simulink model "XMC_DSPLib_Solution_Stage1"  (R2020a)
settings: Solver=VariableStepAuto  StartTime=0.0  StopTime=5000  RelTol=1e-3
PreLoadFcn:
  | CreateFilter;
InitFcn:
  | CreateFilter;
undefined symbols (not defined in the file): cfi, hb1, hb2, hb3, Shift1, Shift2, Shift3, ShiftCF
libraries: ModelComposer x5, dspmlti4 x3, dspsrcs4 x1
settings Model: Creator=oliviert  LastModifiedBy=oliviert

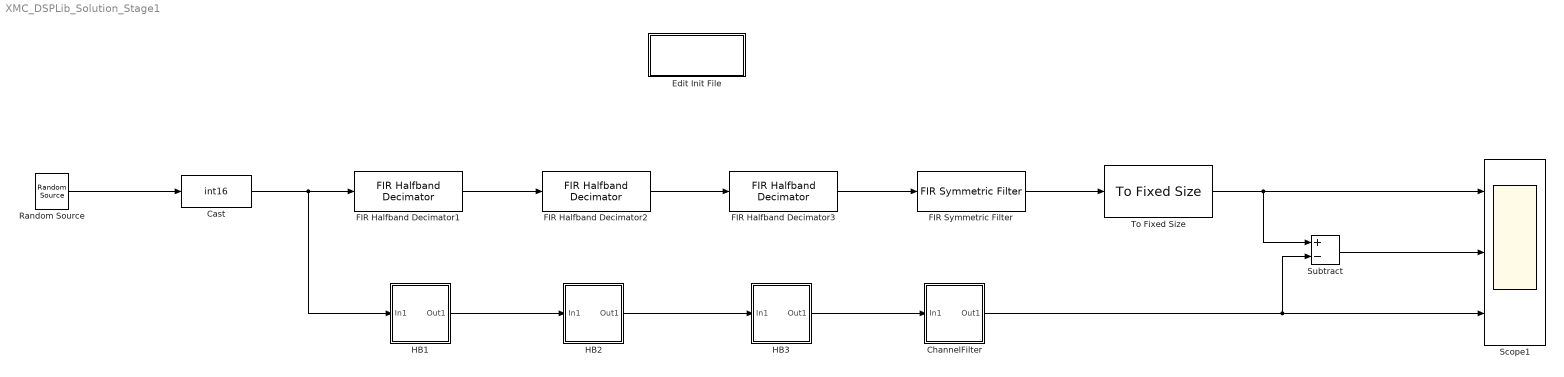
== system XMC_DSPLib_Solution_Stage1 ==
  Cast : DataTypeConversion  OutDataTypeStr=int16
  ChannelFilter : Subsystem  mask{COEFFS=cfi, Shift=ShiftCF}
      mask prompts: COEFFS "Coefficients"; Shift "Final Shift"
  Edit Init File : Subsystem
      settings: OpenFcn=open('CreateFilter.m');
  FIR Halfband Decimator1 : ModelComposer/FIR Halfband Decimator  data_type=cint16  coef_type=int16  use_coeff_reload=off  coeff=hb1_aie  fir_length=31  input_window_size=2048  input_sampling_rate=800  use_casc_length=off  casc_length=1  shift_val=Shift1  rnd_mode=Floor  spec=meta_data_hl_fir_decimate_hb.json
  FIR Halfband Decimator2 : ModelComposer/FIR Halfband Decimator  data_type=cint16  coef_type=int16  use_coeff_reload=off  coeff=hb2_aie  fir_length=31  input_window_size=1024  input_sampling_rate=400  use_casc_length=off  casc_length=1  shift_val=Shift2  rnd_mode=Floor  spec=meta_data_hl_fir_decimate_hb.json
  FIR Halfband Decimator3 : ModelComposer/FIR Halfband Decimator  data_type=cint16  coef_type=int16  use_coeff_reload=off  coeff=hb3_aie  fir_length=31  input_window_size=512  input_sampling_rate=200  use_casc_length=off  casc_length=1  shift_val=Shift3  rnd_mode=Floor  spec=meta_data_hl_fir_decimate_hb.json
  FIR Symmetric Filter : ModelComposer/FIR Symmetric Filter  data_type=cint16  coef_type=int16  use_coeff_reload=off  coeff=cfi_aie  fir_length=length(cfi)  input_window_size=256  input_sampling_rate=100  use_casc_length=off  casc_length=1  shift_val=ShiftCF  rnd_mode=Floor  spec=meta_data_hl_fir_sr_sym.json
  HB1 : Subsystem  mask{COEFFS=hb1, Shift=Shift1}
      mask prompts: COEFFS "Coefficients"; Shift "Final Shift"
  HB2 : Subsystem  mask{COEFFS=hb2, Shift=Shift2}
      mask prompts: COEFFS "Coefficients"; Shift "Final Shift"
  HB3 : Subsystem  mask{COEFFS=hb3, Shift=Shift3}
      mask prompts: COEFFS "Coefficients"; Shift "Final Shift"
  Random Source : dspsrcs4/Random Source  SrcType=Uniform  NormMethod=Ziggurat  CltLength=12  MinVal=-30000  MaxVal=30000  MeanVal=0  VarVal=1  RepMode=Not repeatable  rawSeed=1  IsInherit=off  SampMode=Discrete  SampTime=1  SampFrame=2048  DataType=Double  OutComplex=Complex  OutputFrames=off
  Scope1 : Scope  NumInputPorts=3
  Subtract : Sum  Inputs=+-
  To Fixed Size : ModelComposer/To Fixed Size  OutputSize=256  HasStatusOutput=off
  wires:
  Random Source/1 -> Cast/1
  Cast/1 -> HB1/1(In1), FIR Halfband Decimator1/1
  To Fixed Size/1 -> Subtract/1, Scope1/1
  Subtract/1 -> Scope1/2
  HB1/1(Out1) -> HB2/1(In1)
  FIR Halfband Decimator1/1 -> FIR Halfband Decimator2/1
  FIR Halfband Decimator2/1 -> FIR Halfband Decimator3/1
  FIR Halfband Decimator3/1 -> FIR Symmetric Filter/1
  FIR Symmetric Filter/1 -> To Fixed Size/1
  HB2/1(Out1) -> HB3/1(In1)
  HB3/1(Out1) -> ChannelFilter/1(In1)
  ChannelFilter/1(Out1) -> Subtract/2, Scope1/3

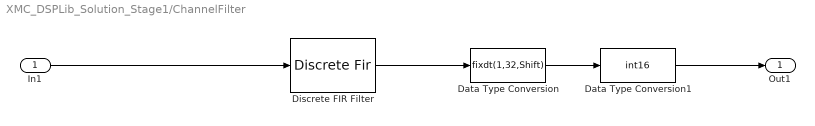
== system XMC_DSPLib_Solution_Stage1/ChannelFilter ==
  In1 : Inport
  Data Type Conversion : DataTypeConversion  OutDataTypeStr=fixdt(1,32,Shift)  ConvertRealWorld=Stored Integer (SI)
  Data Type Conversion1 : DataTypeConversion  OutDataTypeStr=int16  SaturateOnIntegerOverflow=on
  Discrete FIR Filter : DiscreteFir  Coefficients=COEFFS  InputProcessing=Columns as channels (frame based)
  Out1 : Outport
  wires:
  Data Type Conversion/1 -> Data Type Conversion1/1
  In1/1 -> Discrete FIR Filter/1
  Discrete FIR Filter/1 -> Data Type Conversion/1
  Data Type Conversion1/1 -> Out1/1

== system XMC_DSPLib_Solution_Stage1/Edit Init File ==

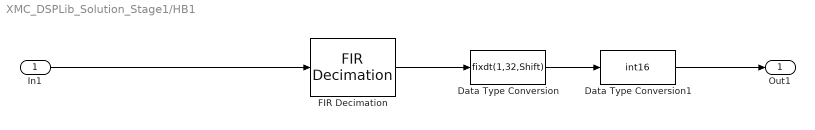
== system XMC_DSPLib_Solution_Stage1/HB1 ==
  In1 : Inport
  Data Type Conversion : DataTypeConversion  OutDataTypeStr=fixdt(1,32,Shift)  ConvertRealWorld=Stored Integer (SI)
  Data Type Conversion1 : DataTypeConversion  OutDataTypeStr=int16  SaturateOnIntegerOverflow=on
  FIR Decimation : dspmlti4/FIR Decimation  FilterSource=Dialog parameters  h=COEFFS  D=2  filtStruct=Direct form  FilterObject=FDECIM  InputProcessing=Columns as channels (frame based)  framing=Enforce single-rate processing  inputOffset=0  outputBufInitCond=0  roundingMode=Floor  overflowMode=off  firstCoeffDataTypeStr=Inherit: Same word length as input  firstCoeffMin=[]  firstCoeffMax=[]  firstCoeffLastDataTypeStr=Inherit: Same word length as input  outputDataTypeStr=Inherit: Same as accumulator  outputMin=[]  outputMax=[]  outputLastDataTypeStr=Inherit: Same as accumulator
  Out1 : Outport
  wires:
  Data Type Conversion1/1 -> Out1/1
  FIR Decimation/1 -> Data Type Conversion/1
  In1/1 -> FIR Decimation/1
  Data Type Conversion/1 -> Data Type Conversion1/1

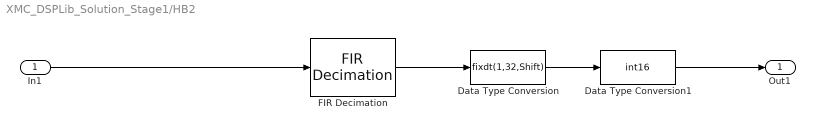
== system XMC_DSPLib_Solution_Stage1/HB2 ==
  In1 : Inport
  Data Type Conversion : DataTypeConversion  OutDataTypeStr=fixdt(1,32,Shift)  ConvertRealWorld=Stored Integer (SI)
  Data Type Conversion1 : DataTypeConversion  OutDataTypeStr=int16  SaturateOnIntegerOverflow=on
  FIR Decimation : dspmlti4/FIR Decimation  FilterSource=Dialog parameters  h=COEFFS  D=2  filtStruct=Direct form  FilterObject=FDECIM  InputProcessing=Columns as channels (frame based)  framing=Enforce single-rate processing  inputOffset=0  outputBufInitCond=0  roundingMode=Floor  overflowMode=off  firstCoeffDataTypeStr=Inherit: Same word length as input  firstCoeffMin=[]  firstCoeffMax=[]  firstCoeffLastDataTypeStr=Inherit: Same word length as input  outputDataTypeStr=Inherit: Same as accumulator  outputMin=[]  outputMax=[]  outputLastDataTypeStr=Inherit: Same as accumulator
  Out1 : Outport
  wires:
  Data Type Conversion/1 -> Data Type Conversion1/1
  In1/1 -> FIR Decimation/1
  FIR Decimation/1 -> Data Type Conversion/1
  Data Type Conversion1/1 -> Out1/1

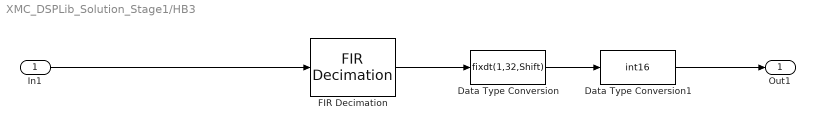
== system XMC_DSPLib_Solution_Stage1/HB3 ==
  In1 : Inport
  Data Type Conversion : DataTypeConversion  OutDataTypeStr=fixdt(1,32,Shift)  ConvertRealWorld=Stored Integer (SI)
  Data Type Conversion1 : DataTypeConversion  OutDataTypeStr=int16  SaturateOnIntegerOverflow=on
  FIR Decimation : dspmlti4/FIR Decimation  FilterSource=Dialog parameters  h=COEFFS  D=2  filtStruct=Direct form  FilterObject=FDECIM  InputProcessing=Columns as channels (frame based)  framing=Enforce single-rate processing  inputOffset=0  outputBufInitCond=0  roundingMode=Floor  overflowMode=off  firstCoeffDataTypeStr=Inherit: Same word length as input  firstCoeffMin=[]  firstCoeffMax=[]  firstCoeffLastDataTypeStr=Inherit: Same word length as input  outputDataTypeStr=Inherit: Same as accumulator  outputMin=[]  outputMax=[]  outputLastDataTypeStr=Inherit: Same as accumulator
  Out1 : Outport
  wires:
  Data Type Conversion1/1 -> Out1/1
  FIR Decimation/1 -> Data Type Conversion/1
  In1/1 -> FIR Decimation/1
  Data Type Conversion/1 -> Data Type Conversion1/1
